simulink model "PIXELdithering_workbench"  (R2020a)
settings: Solver=FixedStepDiscrete  StartTime=0.0  StopTime=10.0  RelTol=1e-3
model workspace (MAT data in the model file):
  led0 = 1
  test = [240 320]
libraries: simulink x55, hdlsllib x29, visionsinks x2, visionzynq_privlib x2, visionhdlutilities x1, visiongeotforms x1, dspvision x1
(part 2 of 2)

== system PIXELdithering_workbench/Modell/P!X3Ldithering/Zeitliches_Dithering_R_G_B1 ==
  note: Pf berechnen.
  note: Wenn Überlauf droht,
      | alten Wert ohne Dithering verwenden.
  note: Bittiefe um 2 Bit
      | reduzieren.
  note: Look-Up-Table um Hf
      | zu berechnen.
  note: Qf
  Farbkanaleingang : Inport
  T+s : Inport  Port=2
  Bit Clear : simulink/Logic and Bit Operations/Bit Clear  iBit=2
      settings: SourceProductBaseCode=SL
  Bit Clear1 : simulink/Logic and Bit Operations/Bit Clear  iBit=3
      settings: SourceProductBaseCode=SL
  Bit Shift : hdlsllib/Logic and Bit Operations/Bit Shift  mode=Shift Left Logical  N=4
  Bit Shift2 : hdlsllib/Logic and Bit Operations/Bit Shift  mode=Shift Right Logical  N=2
  Bitwise Operator : simulink/Logic and Bit Operations/Bitwise Operator  logicop=AND  UseBitMask=on  BitMask=12  BitMaskRealWorld=Stored Integer
  Data Type Conversion2 : DataTypeConversion  OutDataTypeStr=uint8
  Direct Lookup Table (n-D) : LookupNDDirect  Table=[0 1 1 0; 0 0 0 1; 0 0 1 1; 0 0 0 1]  DiagnosticForOutOfRangeInput=Error  TableDataTypeStr=uint8
  HDL Sum2 : Sum  OutDataTypeStr=uint8  SaturateOnIntegerOverflow=on
  Switch1 : Switch  Threshold=240
  Farbkanalausgang_Dithered : Outport
  wires:
  Direct Lookup Table (n-D)/1 -> Bit Shift/1
  Bit Shift/1 -> HDL Sum2/2
  Farbkanaleingang/1 -> Switch1/1, Switch1/2, HDL Sum2/1, Data Type Conversion2/1
  Bit Clear/1 -> Bit Clear1/1
  Bit Clear1/1 -> Farbkanalausgang_Dithered/1
  Bitwise Operator/1 -> Bit Shift2/1
  Bit Shift2/1 -> Direct Lookup Table (n-D)/2
  Data Type Conversion2/1 -> Bitwise Operator/1
  HDL Sum2/1 -> Switch1/3
  Switch1/1 -> Bit Clear/1
  T+s/1 -> Direct Lookup Table (n-D)/1

== system PIXELdithering_workbench/Modell/P!X3Ldithering/Zeitliches_Dithering_R_G_B2 ==
  note: Pf berechnen.
  note: Wenn Überlauf droht,
      | alten Wert ohne Dithering verwenden.
  note: Bittiefe um 2 Bit
      | reduzieren.
  note: Look-Up-Table um Hf
      | zu berechnen.
  note: Qf
  Farbkanaleingang : Inport
  T+s : Inport  Port=2
  Bit Clear : simulink/Logic and Bit Operations/Bit Clear  iBit=2
      settings: SourceProductBaseCode=SL
  Bit Clear1 : simulink/Logic and Bit Operations/Bit Clear  iBit=3
      settings: SourceProductBaseCode=SL
  Bit Shift : hdlsllib/Logic and Bit Operations/Bit Shift  mode=Shift Left Logical  N=4
  Bit Shift2 : hdlsllib/Logic and Bit Operations/Bit Shift  mode=Shift Right Logical  N=2
  Bitwise Operator : simulink/Logic and Bit Operations/Bitwise Operator  logicop=AND  UseBitMask=on  BitMask=12  BitMaskRealWorld=Stored Integer
  Data Type Conversion2 : DataTypeConversion  OutDataTypeStr=uint8
  Direct Lookup Table (n-D) : LookupNDDirect  Table=[0 1 1 0; 0 0 0 1; 0 0 1 1; 0 0 0 1]  DiagnosticForOutOfRangeInput=Error  TableDataTypeStr=uint8
  HDL Sum2 : Sum  OutDataTypeStr=uint8  SaturateOnIntegerOverflow=on
  Switch1 : Switch  Threshold=240
  Farbkanalausgang_Dithered : Outport
  wires:
  Direct Lookup Table (n-D)/1 -> Bit Shift/1
  Bit Shift/1 -> HDL Sum2/2
  Farbkanaleingang/1 -> Switch1/1, Switch1/2, HDL Sum2/1, Data Type Conversion2/1
  Bit Clear/1 -> Bit Clear1/1
  Bit Clear1/1 -> Farbkanalausgang_Dithered/1
  Bitwise Operator/1 -> Bit Shift2/1
  Bit Shift2/1 -> Direct Lookup Table (n-D)/2
  Data Type Conversion2/1 -> Bitwise Operator/1
  HDL Sum2/1 -> Switch1/3
  Switch1/1 -> Bit Clear/1
  T+s/1 -> Direct Lookup Table (n-D)/1

== matlab function PIXELdithering_workbench/Modell/P!X3Ldithering/Raeumliches_Dithering_G/MATLAB Function ==
  data: x input; He output; y input; Xmod3 input; Ymod3 input; Qe input
function He = fcn(x, y, Xmod3, Ymod3, Qe)

if Xmod3 < 2 && Ymod3 < 2
    Bereichsel = 0;
elseif Xmod3 > 1 && Ymod3 < 2
    Bereichsel = 1;
elseif Xmod3 > 2 && Ymod3 > 2
    Bereichsel = 2;
else 
    Bereichsel = 3;
end

% He in Abhängigkeit der Positon. Ergibt mit dem zeitlichen Dithering eine
% Struktur, bei der die Helligkeit bei 4x4 Pixel konstant bleibt. 
%   
% Bereichsel|    Qe  0    1     2     3
%-----------------------------------------------
%           |       x  
%           |       0 1
%           |    
%     0     |  y 0  0 0   0 0   0 1   1 1
%           |    1  0 0   1 0   1 0   0 1 
%           |
%     1     |       0 0   1 0   1 0   1 1
%           |       0 0   0 0   0 1   1 0 
%           |        
%     2     |       0 0   0 1   0 1   1 0
%           |       0 0   0 0   1 0   1 1
%           |       
%     3     |       0 0   0 0   1 0   1 1
%           |       0 0   0 1   0 1   1 0
%

He_Matrix =  cat(4,cat(3, [0 0; 0 0], [0 0; 0 0], [0 0; 0 0],[0 0; 0 0]),cat(3,[0 0; 1 0], [1 0; 0 0], [0 1; 0 0], [0 0; 0 1]), cat(3,[0 1; 1 0], [1 0; 0 1], [0 1; 1 0], [1 0; 0 1]), cat(3, [1 1; 0 1], [1 1; 1 0], [1 0; 1 1], [1 1; 1 0]));
He = cast(He_Matrix(x+1, y+1, Bereichsel+1, Qe+1),'uint8'); % Cast auf uint8 da sonst Ausgabe als Floating-Point, 
                                                            % das vom HDL-Coder nicht unterstüzt wird.

== matlab function PIXELdithering_workbench/Modell/P!X3Ldithering/Raeumliches_Dithering_R_B/MATLAB Function ==
  data: x input; He output; y input; Xmod3 input; Ymod3 input; Qe input
function He = fcn(x, y, Xmod3, Ymod3, Qe)

if Xmod3 < 2 && Ymod3 < 2
    Bereichsel = 0;
elseif Xmod3 > 1 && Ymod3 < 2
    Bereichsel = 1;
elseif Xmod3 > 2 && Ymod3 > 2
    Bereichsel = 2;
else 
    Bereichsel = 3;
end

% He in Abhängigkeit der Positon. Ergibt mit dem zeitlichen Dithering eine
% Struktur, bei der die Helligkeit bei 4x4 Pixel konstant bleibt. 
%   
% Bereichsel|    Qe  0    1     2     3
%-----------------------------------------------
%           |       x  
%           |       0 1
%           |    
%     0     |  y 0  0 0   0 1   1 0   1 0
%           |    1  0 0   0 0   0 1   1 1 
%           |
%     1     |       0 0   0 0   0 1   1 1
%           |       0 0   0 1   1 0   1 0 
%           |        
%     2     |       0 0   0 0   1 0   1 1
%           |       0 0   1 0   0 1   0 1
%           |       
%     3     |       0 0   1 0   0 1   0 1
%           |       0 0   0 0   1 0   1 1
%

He_Matrix = cat(4,cat(3, [0 0; 0 0], [0 0; 0 0], [0 0; 0 0],[0 0; 0 0]),cat(3,[0 1; 0 0], [0 0; 0 1], [0 0; 1 0], [1 0; 0 0]), cat(3,[1 0; 0 1], [0 1; 1 0], [1 0; 0 1], [0 1; 1 0]), cat(3, [1 0; 1 1], [1 1; 1 0], [1 1; 0 1], [0 1; 1 1]));
He = cast(He_Matrix(x+1, y+1, Bereichsel+1, Qe+1),'uint8'); % Cast auf uint8 da sonst Ausgabe als Floating-Point, 
                                                            % das vom HDL-Coder nicht unterstüzt wird.

== matlab function PIXELdithering_workbench/Modell/P!X3Ldithering/Raeumliches_Dithering_R_B2/MATLAB Function ==
  data: x input; He output; y input; Xmod3 input; Ymod3 input; Qe input
function He = fcn(x, y, Xmod3, Ymod3, Qe)

if Xmod3 < 2 && Ymod3 < 2
    Bereichsel = 0;
elseif Xmod3 > 1 && Ymod3 < 2
    Bereichsel = 1;
elseif Xmod3 > 2 && Ymod3 > 2
    Bereichsel = 2;
else 
    Bereichsel = 3;
end

% He in Abhängigkeit der Positon. Ergibt mit dem zeitlichen Dithering eine
% Struktur, bei der die Helligkeit bei 4x4 Pixel konstant bleibt. 
%   
% Bereichsel|    Qe  0    1     2     3
%-----------------------------------------------
%           |       x  
%           |       0 1
%           |    
%     0     |  y 0  0 0   0 1   1 0   1 0
%           |    1  0 0   0 0   0 1   1 1 
%           |
%     1     |       0 0   0 0   0 1   1 1
%           |       0 0   0 1   1 0   1 0 
%           |        
%     2     |       0 0   0 0   1 0   1 1
%           |       0 0   1 0   0 1   0 1
%           |       
%     3     |       0 0   1 0   0 1   0 1
%           |       0 0   0 0   1 0   1 1
%

He_Matrix = cat(4,cat(3, [0 0; 0 0], [0 0; 0 0], [0 0; 0 0],[0 0; 0 0]),cat(3,[0 1; 0 0], [0 0; 0 1], [0 0; 1 0], [1 0; 0 0]), cat(3,[1 0; 0 1], [0 1; 1 0], [1 0; 0 1], [0 1; 1 0]), cat(3, [1 0; 1 1], [1 1; 1 0], [1 1; 0 1], [0 1; 1 1]));
He = cast(He_Matrix(x+1, y+1, Bereichsel+1, Qe+1),'uint8'); % Cast auf uint8 da sonst Ausgabe als Floating-Point, 
                                                            % das vom HDL-Coder nicht unterstüzt wird.

== matlab function PIXELdithering_workbench/Modell/MATLAB Function ==
  data: x input; z output; y input; Xmod3 input; Ymod3 input; E input
function z = fcn(x, y,Xmod3,Ymod3, E)

if Xmod3 < 2 && Ymod3 < 2
    t = 0;
elseif Xmod3 > 1 && Ymod3 < 2
    t = 1;
elseif Xmod3 > 2 && Ymod3 > 2
    t = 2;
else 
    t = 3;
end
A = cat(4,cat(3, [0 0; 0 0], [0 0; 0 0], [0 0; 0 0],[0 0; 0 0]),cat(3,[0 0; 1 0], [1 0; 0 0], [0 1; 0 0], [0 0; 0 1]), cat(3,[0 1; 1 0], [1 0; 0 1], [0 1; 1 0], [1 0; 0 1]), cat(3, [1 1; 0 1], [1 1; 1 0], [1 0; 1 1], [1 1; 1 0]));
z = cast(A(x+1, y+1, t+1, E+1),'uint8');
